simulink model "TrimFandM"  (R2020a)
settings: Solver=VariableStepAuto  StartTime=0.0  StopTime=10.0  RelTol=1e-3
values from neighbouring files (symbols this model uses):
  D = (1/2)*rho*velmag^2*refarea*cD    [AFDTrim.m]    (also in ForceMoment.m)
  nfs = AFDCtrlDesign(nfs)    [AFDSimInit.m]    (also in AFDSimInitDatcom.m = PlaneData('SI'); TransferFunction.m = PlaneData('SI'))
undefined symbols (not defined in the file or in its folder): TrimTrial
libraries: NFSModelsLibrary x1
settings Model: SimulationMode=accelerator  Creator=AHKh  LastModifiedBy=AHKh
settings DataIOCC: ReturnWorkspaceOutputs=off
settings DebuggingCC: ArithmeticOperatorsInVariantConditions=warning
settings SFSimCC: SimUseLocalCustomCode=off  CustomCodeUndefinedFunction=UseInterfaceOnly
settings RTWCC: RTWUseLocalCustomCode=off

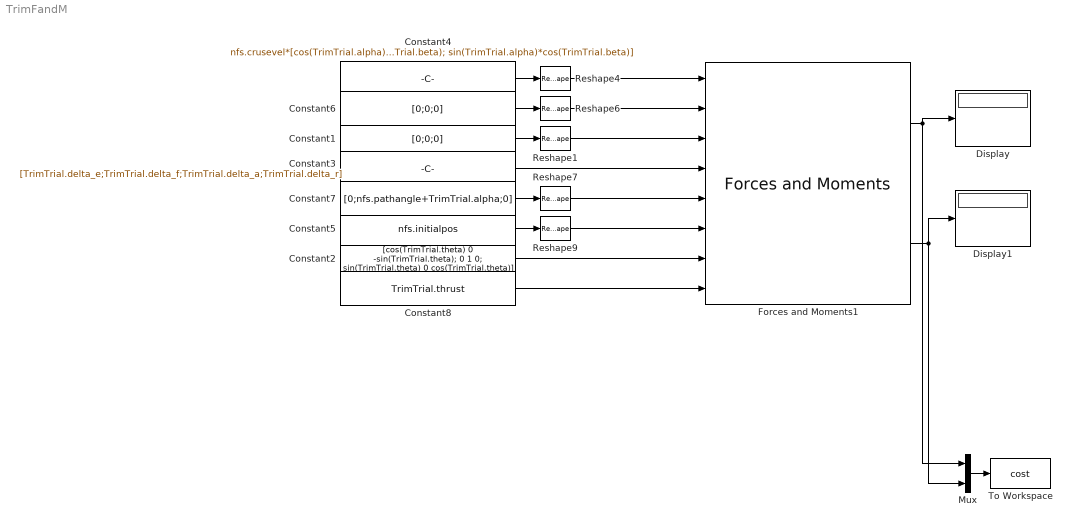
== system TrimFandM ==
  Constant1 : Constant  Value=[0;0;0]
  Constant2 : Constant  Value=[cos(TrimTrial.theta) 0 -sin(TrimTrial.theta); 0 1 0; sin(TrimTrial.theta) 0 cos(TrimTrial.theta)]
  Constant3 : Constant  Value=[TrimTrial.delta_e;TrimTrial.delta_f;TrimTrial.delta_a;TrimTrial.delta_r]
  Constant4 : Constant  Value=nfs.crusevel*[cos(TrimTrial.alpha)*cos(TrimTrial.beta); sin(TrimTrial.beta); sin(TrimTrial.alpha)*cos(TrimTrial.beta)]
  Constant5 : Constant  Value=nfs.initialpos
  Constant6 : Constant  Value=[0;0;0]
  Constant7 : Constant  Value=[0;nfs.pathangle+TrimTrial.alpha;0]
  Constant8 : Constant  Value=TrimTrial.thrust
  Display : Display
  Display1 : Display
  Forces and Moments1 : NFSModelsLibrary/Forces and Moments  SystemSampleTime=-1  Latency=0  AutoFrameSizeCalculation=off
  Mux : Mux  Inputs=2
  Reshape{1,4,6..7,9} (5 alike) : Reshape  OutputDimensionality=Column vector (2-D)
  To Workspace : ToWorkspace  VariableName=cost  SaveFormat=Timeseries  SampleTime=-1
  wires:
  Constant6/1 -> Reshape6/1
  Reshape6/1 -> Forces and Moments1/2
  Constant1/1 -> Reshape1/1
  Reshape1/1 -> Forces and Moments1/3
  Constant4/1 -> Reshape4/1
  Reshape4/1 -> Forces and Moments1/1
  Constant7/1 -> Reshape7/1
  Reshape7/1 -> Forces and Moments1/5
  Constant5/1 -> Reshape9/1
  Reshape9/1 -> Forces and Moments1/6
  Constant2/1 -> Forces and Moments1/7
  Constant3/1 -> Forces and Moments1/4
  Forces and Moments1/1 -> Display/1, Mux/1
  Forces and Moments1/2 -> Display1/1, Mux/2
  Mux/1 -> To Workspace/1
  Constant8/1 -> Forces and Moments1/8
